simulink model "msd"  (R2021a)
settings: Solver=VariableStepAuto  StartTime=0.0  StopTime=100  RelTol=1e-3
values from neighbouring files (symbols this model uses):
  b = 1.2    [mpcEffort.m]
  k = 1    [mpcEffort.m]
  m = 1    [mpcEffort.m]
settings Model: Creator=jamagola  LastModifiedBy=jamagola

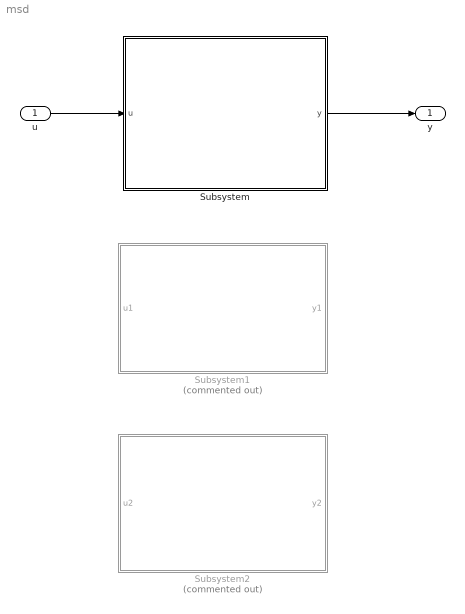
== system msd ==
  u : Inport
  Subsystem : Subsystem
  Subsystem1 : Subsystem  Commented=on
  Subsystem2 : Subsystem  Commented=on
  y : Outport
  wires:
  u/1 -> Subsystem/1(u)
  Subsystem/1(y) -> y/1

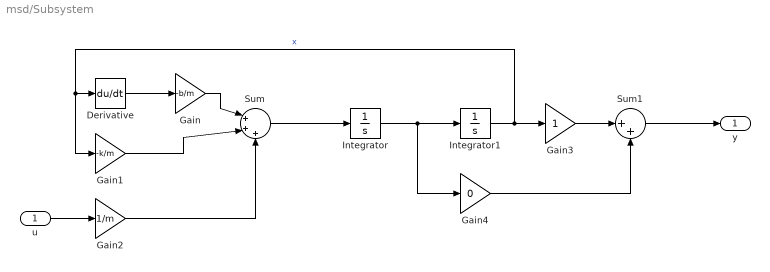
== system msd/Subsystem ==
  u : Inport
  Derivative : Derivative
  Gain : Gain  Gain=-b/m
  Gain1 : Gain  Gain=-k/m
  Gain2 : Gain  Gain=1/m
  Gain3 : Gain
  Gain4 : Gain  Gain=0
  Integrator : Integrator
  Integrator1 : Integrator
  Sum : Sum  Inputs=|+++
  Sum1 : Sum  Inputs=|++
  y : Outport
  wires:
  u/1 -> Gain2/1
  Sum1/1 -> y/1
  Integrator/1 -> Gain4/1, Integrator1/1
  Derivative/1 -> Gain/1
  Sum/1 -> Integrator/1
  Gain4/1 -> Sum1/2
  Gain/1 -> Sum/1
  Integrator1/1 -> Derivative/1, Gain1/1, Gain3/1  "x"
  Gain3/1 -> Sum1/1
  Gain1/1 -> Sum/2
  Gain2/1 -> Sum/3

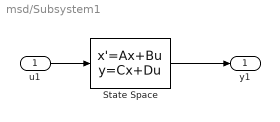
== system msd/Subsystem1 ==
  u1 : Inport
  State Space : StateSpace  A=[0 1; -k/m -b/m]  B=[0; 1/m]  C=[1 0]  D=0  InitialCondition=[0;0]
  y1 : Outport
  wires:
  u1/1 -> State Space/1
  State Space/1 -> y1/1

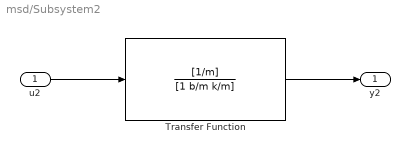
== system msd/Subsystem2 ==
  u2 : Inport
  Transfer Function : TransferFcn  Numerator=[1/m]  Denominator=[1 b/m k/m]
  y2 : Outport
  wires:
  u2/1 -> Transfer Function/1
  Transfer Function/1 -> y2/1
